simulink model "s_servo_speed_cntrl2"  (R2019a)
settings: Solver=ode4  StartTime=0.0  StopTime=5  FixedStep=0.001  RelTol=1e-3  AbsTol=1e-6  EnableMultiTasking=on
values from neighbouring files (symbols this model uses):
  a = 1    [setup_servo_speed_cntrl2.m]
  bsp = 0    [setup_servo_speed_cntrl2.m]
  K = 10    [setup_servo_speed_cntrl2.m]
  Kc = 0    [setup_servo_speed_cntrl2.m]
  ki = 0    [setup_servo_speed_cntrl2.m]
  kp = 0    [setup_servo_speed_cntrl2.m]
  T = 1    [setup_servo_speed_cntrl2.m]
  tau = 0.1    [setup_servo_speed_cntrl2.m]
libraries: simulink x2, quarc_library x1
settings Model: ExtModeTrigDuration=10000  Creator=MLevis  LastModifiedBy=pmartin
settings SolverCC: AutoScaleAbsTol=off  PositivePriorityOrder=on
settings DataIOCC: SaveFormat=Array  SignalLoggingSaveFormat=ModelDataLogs  ReturnWorkspaceOutputs=off
settings OptimizationCC: BlockReduction=off  BooleanDataType=off  OptimizeBlockIOStorage=off  BufferReuse=off  GlobalBufferReuse=off  ExpressionFolding=off  ExpressionDepthLimit=2147483647  LocalBlockOutputs=off  InitFltsAndDblsToZero=on  OptimizeDataStoreBuffers=off  BusAssignmentInplaceUpdate=off
settings DebuggingCC: SaveWithParameterizedLinksMsg=none  UnderspecifiedInitializationDetection=Classic  MergeDetectMultiDrivingBlocksExec=none  SignalResolutionControl=TryResolveAllWithWarning  MultiTaskDSMMsg=warning  MultiTaskCondExecSysMsg=none  FcnCallInpInsideContextMsg=warning  StateNameClashWarn=warning  SFUnexpectedBacktrackingDiag=warning  SFNoUnconditionalDefaultTransitionDiag=warning  SFExecutionAtInitializationDiag=none  ArithmeticOperatorsInVariantConditions=warning
settings HardwareCC: ProdBitPerPointer=32  ProdBitPerSizeT=32  ProdBitPerPtrDiffT=32  ProdLargestAtomicFloat=None  ProdIntDivRoundTo=Undefined  ProdEndianess=Unspecified  ProdWordSize=32  ProdHWDeviceType=32-bit Generic  TargetHWDeviceType=32-bit Generic
settings ModelReferenceCC: PropagateSignalLabelsOutOfModel=off
settings RTWCC: SystemTargetFile=quarc_win64.tlc  TemplateMakefile=quarc_default_tmf  Description=QUARC Win64 Target
settings CodeAppCC: StateflowObjectComments=on
settings STFCustomTargetCC: TargetPreCompLibLocation=C:\PROGRA~3\QUARC\lib\2019a\win64\release  ConcurrentExecutionCompliant=on  SystemTargetFile=quarc_win64.tlc
settings GRTTargetCC: TargetPreCompLibLocation=C:\PROGRA~3\QUARC\lib\2019a\win64\release  TargetLangStandard=C89/C90 (ANSI)  ParMdlRefBuildCompliant=off  CompOptLevelCompliant=off  CombineOutputUpdateFcns=off  MatFileLogging=off  CPPClassGenCompliant=off  GRTInterface=on  UseToolchainInfoCompliant=off  ExtMode=on  ExtModeMexFile=quarc_comm
settings ConfigComp: CovMetricSettings=dw  CovHtmlReporting=on  CovSaveCumulativeToWorkspaceVar=on  CovSaveSingleToWorkspaceVar=on

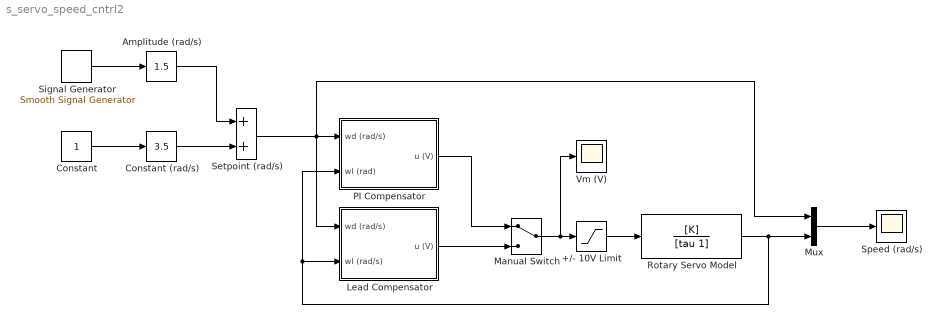
== system s_servo_speed_cntrl2 ==
  +/- 10V Limit : Saturate  UpperLimit=10  LowerLimit=-10
  Amplitude (rad/s) : simulink/Math Operations/Slider Gain  gain=1.5  low=0  high=10
  "Constant " : Constant
  Constant (rad/s) : simulink/Math Operations/Slider Gain  gain=3.5  low=0  high=20
  Lead Compensator : Subsystem
  Manual Switch : ManualSwitch
  Mux : Mux  Inputs=2
  PI Compensator : Subsystem
  Rotary Servo Model : TransferFcn  Numerator=[K]  Denominator=[tau 1]
  Setpoint (rad/s) : Sum
  Signal Generator : quarc_library/Sources/Signals/Smooth Signal Generator  signal_type=Square  source=Internal (dialog parameters)  amplitude=1  frequency=0.4  initial_phase=0  sample_time=qc_get_step_size  output_cos=off
      settings: SourceProductName=QUARC Targets
  Speed (rad/s) : Scope
  Vm (V) : Scope
  wires:
  Setpoint (rad/s)/1 -> Mux/1, PI Compensator/1(wd (rad/s)), Lead Compensator/1(wd (rad/s))
  Manual Switch/1 -> Vm (V)/1, +/- 10V Limit/1
  Mux/1 -> Speed (rad/s)/1
  Lead Compensator/1(u (V)) -> Manual Switch/2
  PI Compensator/1(u (V)) -> Manual Switch/1
  Signal Generator/1 -> Amplitude (rad/s)/1
  Amplitude (rad/s)/1 -> Setpoint (rad/s)/1
  "Constant "/1 -> Constant (rad/s)/1
  Constant (rad/s)/1 -> Setpoint (rad/s)/2
  Rotary Servo Model/1 -> Mux/2, Lead Compensator/2(wl (rad/s)), PI Compensator/2(wl (rad))
  +/- 10V Limit/1 -> Rotary Servo Model/1

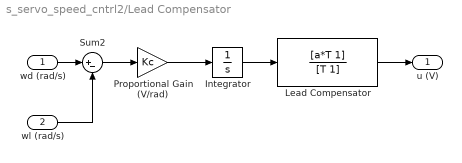
== system s_servo_speed_cntrl2/Lead Compensator ==
  wd (rad/s) : Inport
  wl (rad/s) : Inport  Port=2
  Integrator : Integrator
  Lead Compensator : TransferFcn  Numerator=[a*T 1]  Denominator=[T 1]
  Proportional Gain (V/rad) : Gain  Gain=Kc
  Sum2 : Sum  Inputs=|+-
  u (V) : Outport
  wires:
  Lead Compensator/1 -> u (V)/1
  Proportional Gain (V/rad)/1 -> Integrator/1
  Integrator/1 -> Lead Compensator/1
  Sum2/1 -> Proportional Gain (V/rad)/1
  wd (rad/s)/1 -> Sum2/1
  wl (rad/s)/1 -> Sum2/2

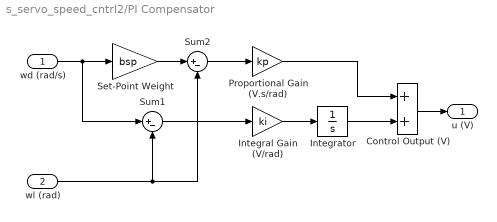
== system s_servo_speed_cntrl2/PI Compensator ==
  wd (rad/s) : Inport
  wl (rad) : Inport  Port=2
  Control Output (V) : Sum
  Integral Gain (V/rad) : Gain  Gain=ki
  Integrator : Integrator  UpperSaturationLimit=10  LowerSaturationLimit=-10
  Proportional Gain (V.s/rad) : Gain  Gain=kp
  Set-Point Weight : Gain  Gain=bsp
  Sum1 : Sum  Inputs=|+-
  Sum2 : Sum  Inputs=|+-
  u (V) : Outport
  wires:
  Sum1/1 -> Integral Gain (V/rad)/1
  Integral Gain (V/rad)/1 -> Integrator/1
  Integrator/1 -> Control Output (V)/2
  Proportional Gain (V.s/rad)/1 -> Control Output (V)/1
  Set-Point Weight/1 -> Sum2/1
  Sum2/1 -> Proportional Gain (V.s/rad)/1
  wd (rad/s)/1 -> Set-Point Weight/1, Sum1/1
  Control Output (V)/1 -> u (V)/1
  wl (rad)/1 -> Sum1/2, Sum2/2
